simulink model "Vorlage_Gesamtanlage"  (R2022a)
settings: Solver=ode5  StartTime=0.0  StopTime=200  FixedStep=0.01  MaxStep=1  MinStep=0.005  RelTol=1e-3  AbsTol=10  EnableMultiTasking=on
values from neighbouring files (symbols this model uses):
  A = 5    [Parameter.m]
  Flaschengroesse = 10    [Parameter.m]
  I = 0.5    [Parameter.m]
  igetr = 1080    [Parameter.m]
  K = 8    [Parameter.m]
  MaxFlaschen = 25    [Parameter.m]
  MRK = 1    [Parameter.m]
  numA = 0    [Parameter.m]
  PassSilo1 = 1    [Parameter.m]
  PassSilo2 = 1    [Parameter.m]
  PHI = 0.001    [Parameter.m]
  Ra = 40    [Parameter.m]
  SizeSilo1 = 15    [Parameter.m]
  SizeSilo2 = 15    [Parameter.m]
  U = 24    [Parameter.m]
  v_band_abfuhr_set = 2    [Parameter.m]
  v_band_arbeit_set = 30    [Parameter.m]
  v_band_zufuhr_set = 10    [Parameter.m]
  v_umsetzer_greifer_set = 400    [Parameter.m]
  v_umsetzer_set = 80    [Parameter.m]
  v_ve1_set = 400    [Parameter.m]
  v_ve2_set = 400    [Parameter.m]
undefined symbols (not defined in the file or in its folder): Limits
libraries: simulink x94
(part 3 of 3)

== system Vorlage_Gesamtanlage/Abfüllanlage/Flaschen_data/Flaschenstarter/in_Flaschenzähler ==
  Signal : Inport
  Constant : Constant
  Constant1 : Constant  Value=0
  Logical Operator : Logic  AllPortsSameDT=off
  Memory : Memory
  Memory1 : Memory
  Relational Operator : RelationalOperator  Operator===  InputSameDT=off
  Relational Operator1 : RelationalOperator  Operator===  InputSameDT=off
  Sum : Sum  Inputs=|++  OutDataTypeStr=uint16  SaturateOnIntegerOverflow=on
  Rising Edge : Outport
  Count : Outport  Port=2
  wires:
  Signal/1 -> Memory/1, Relational Operator/2
  Constant/1 -> Relational Operator/1
  Relational Operator/1 -> Logical Operator/1
  Constant1/1 -> Relational Operator1/2
  Memory/1 -> Relational Operator1/1
  Relational Operator1/1 -> Logical Operator/2
  Logical Operator/1 -> Sum/1, Rising Edge/1
  Memory1/1 -> Sum/2
  Sum/1 -> Count/1, Memory1/1

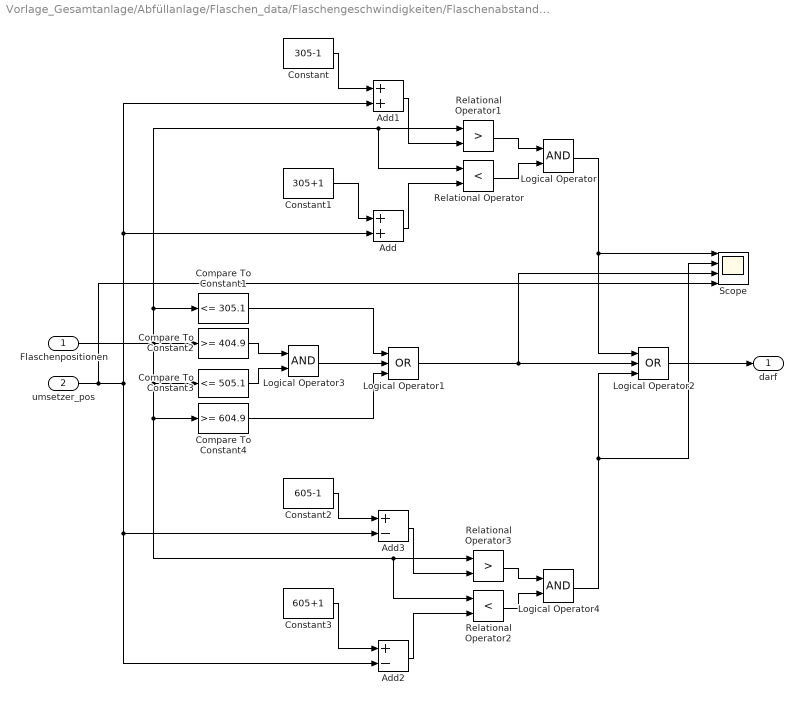
== system Vorlage_Gesamtanlage/Abfüllanlage/Flaschen_data/Flaschengeschwindigkeiten/Flaschenabstandsüberwachung/Umsetzer darf mitnehmen ==
  Flaschenpositionen : Inport
  umsetzer_pos : Inport  Port=2
  Add : Sum
  Add1 : Sum
  Add2 : Sum  Inputs=+-
  Add3 : Sum  Inputs=+-
  Compare To Constant1 : simulink/Logic and Bit Operations/Compare To Constant  relop=<=  const=305.1  OutDataTypeStr=uint8  ZeroCross=off
  Compare To Constant2 : simulink/Logic and Bit Operations/Compare To Constant  relop=>=  const=404.9  OutDataTypeStr=uint8  ZeroCross=off
  Compare To Constant3 : simulink/Logic and Bit Operations/Compare To Constant  relop=<=  const=505.1  OutDataTypeStr=uint8  ZeroCross=off
  Compare To Constant4 : simulink/Logic and Bit Operations/Compare To Constant  relop=>=  const=604.9  OutDataTypeStr=uint8  ZeroCross=off
  Constant : Constant  Value=305-1
  Constant1 : Constant  Value=305+1
  Constant2 : Constant  Value=605-1
  Constant3 : Constant  Value=605+1
  Logical Operator : Logic  AllPortsSameDT=off  OutDataTypeStr=boolean
  Logical Operator1 : Logic  Operator=OR  Inputs=3  AllPortsSameDT=off  OutDataTypeStr=boolean
  Logical Operator2 : Logic  Operator=OR  Inputs=3  AllPortsSameDT=off  OutDataTypeStr=boolean
  Logical Operator3 : Logic  AllPortsSameDT=off  OutDataTypeStr=boolean
  Logical Operator4 : Logic  AllPortsSameDT=off  OutDataTypeStr=boolean
  Relational Operator : RelationalOperator  Operator=<  OutDataTypeStr=boolean  InputSameDT=off
  Relational Operator1 : RelationalOperator  Operator=>  OutDataTypeStr=boolean  InputSameDT=off
  Relational Operator2 : RelationalOperator  Operator=<  OutDataTypeStr=boolean  InputSameDT=off
  Relational Operator3 : RelationalOperator  Operator=>  OutDataTypeStr=boolean  InputSameDT=off
  Scope : Scope  NumInputPorts=4
  darf : Outport
  wires:
  Logical Operator2/1 -> darf/1
  Logical Operator1/1 -> Logical Operator2/2, Scope/3
  Compare To Constant1/1 -> Logical Operator1/1
  Logical Operator/1 -> Logical Operator2/1, Scope/1
  Constant/1 -> Add1/1
  Add1/1 -> Relational Operator1/2
  Relational Operator1/1 -> Logical Operator/1
  Relational Operator/1 -> Logical Operator/2
  Add/1 -> Relational Operator/2
  Constant1/1 -> Add/1
  Compare To Constant2/1 -> Logical Operator3/1
  Compare To Constant3/1 -> Logical Operator3/2
  Logical Operator3/1 -> Logical Operator1/2
  Compare To Constant4/1 -> Logical Operator1/3
  Logical Operator4/1 -> Logical Operator2/3, Scope/2
  Constant2/1 -> Add3/1
  Add3/1 -> Relational Operator3/2
  Relational Operator3/1 -> Logical Operator4/1
  Relational Operator2/1 -> Logical Operator4/2
  Add2/1 -> Relational Operator2/2
  Constant3/1 -> Add2/1
  umsetzer_pos/1 -> Add2/2, Add3/2, Add/2, Add1/2, Scope/4
  Flaschenpositionen/1 -> Compare To Constant2/1, Compare To Constant3/1, Compare To Constant4/1, Relational Operator3/1, Relational Operator2/1, Compare To Constant1/1, Relational Operator1/1, Relational Operator/1

== stateflow chart Vorlage_Gesamtanlage/Abfüllanlage/Drehscheibe/Sensor ==
  state Start
    en: beep = 0;
  state Beep
    en: beep=1;
  (default) -> Start
  Start -> Beep : [ml.mod(winkel, 90) <=2 | ml.mod(winkel, 90) >=88]
  Beep -> Start : [ml.mod(winkel, 90) >2 && ml.mod(winkel, 90) <88]
  data: winkel input double; beep output boolean

== stateflow chart Vorlage_Gesamtanlage/Abfüllanlage/Fehlererkennung/Volle Flasche zum Teller zurück/Chart ==
  state Greife_Flasche_Teller
    entry: error = 0;
  state Oeffne_Greifer_Band
  state Warte_auf_VE2
  state Volle_Flasche_gegriffen
  state Greifer_gestartet
    entry: error = 1;
  state Flasche_weg
  (default) -> Greife_Flasche_Teller
  Flasche_weg -> Greife_Flasche_Teller
  Greife_Flasche_Teller -> Oeffne_Greifer_Band : [I_teller_behaelter_hinten == 1 && i_greifer_zu == 1 && i_umsetz_teller == 1]
  Oeffne_Greifer_Band -> Warte_auf_VE2 : [i_greifer_auf == 1 && i_umsetz_band == 1]
  Volle_Flasche_gegriffen -> Greifer_gestartet [order 1] : [o_umsetz_teller==1]
  Warte_auf_VE2 -> Volle_Flasche_gegriffen [order 2] : [i_greifer_zu == 1]
  Warte_auf_VE2 -> Flasche_weg [order 1] : [i_ve2_herein == 1]
  Volle_Flasche_gegriffen -> Flasche_weg [order 2] : after(5,sec)
  data: I_teller_behaelter_hinten input; i_greifer_zu input; i_umsetz_teller input; i_greifer_auf input; i_umsetz_band input; i_ve2_herein input; error output; o_umsetz_teller input

== stateflow chart Vorlage_Gesamtanlage/Steuerung ==
  state Intelligenz [parallel]
    settings: executionOrder=1
    state Flasche_bewegen [parallel]
      settings: executionOrder=1
      state Initiation
      state Baender_an
        en: send(Arbeitsband_an,Baender);
      state Leere_Flasche_loslassen
        en: send(ums_greifer_auf,Umsetzer)
      state Leere_Flasche_greifen
        en: send(ums_Flasche_greifen,Umsetzer)
      state Umsetzer_zu_Band
        en: send(ums_zu_band,Umsetzer);
      state Leere_Flasche_zu_Teller_umsetzen
        en: send(ums_zu_teller,Umsetzer)
      state Vereineinzeler_1_oeffnen
        en: send(ve1_oeffnen,VE1_2)
        %Dann Leere Flasche durchgehen
      state Leere_Flasche_befuellen
        en: send(silos_oeffnen,Silos)
      state Gefuellte_Flasche_greifen
        en: send(ums_Flasche_greifen,Umsetzer)
      state Gefuellte_Flasche_zu_Band_umsetzen
        en: send(ums_zu_band,Umsetzer)
      state Gefuellte_Flasche_loslassen
        en: send(ums_greifer_auf,Umsetzer)
      state Vereinzeler_2_oeffnen
        en: send(ve2_oeffnen,VE1_2)
        %Dann Gefuellte Flasche weggehne
      state Teller_drehen
        en: send(teller_drehen,Teller)
      state Teller_ausgerichtet
        en: send(teller_ausg,Teller)
        en: send(check,Flasche_voll_check)
      (default) -> Intelligenz.Flasche_bewegen.Initiation
      Intelligenz.Flasche_bewegen.Initiation -> Baender_an
      Baender_an -> Intelligenz.Flasche_bewegen.Umsetzer_zu_Band : [i_umsetzer[3] == 1]
      Intelligenz.Flasche_bewegen.Teller_ausgerichtet -> Intelligenz.Flasche_bewegen.Umsetzer_zu_Band [order 1] : [i_silo[2] == 0 && i_teller[2] == 0]
      Intelligenz.Flasche_bewegen.Leere_Flasche_greifen -> Leere_Flasche_zu_Teller_umsetzen : [i_umsetzer[4] == 1]
      Vereineinzeler_1_oeffnen -> Intelligenz.Flasche_bewegen.Leere_Flasche_greifen : [i_vereinzeler[6] == 1]
      Leere_Flasche_zu_Teller_umsetzen -> Leere_Flasche_loslassen : [i_umsetzer[2] == 1]
      Intelligenz.Flasche_bewegen.Umsetzer_zu_Band -> Vereineinzeler_1_oeffnen : [i_vereinzeler[5] == 1 && i_vereinzeler[6] == 0 && i_teller[2] == 0 && i_umsetzer[1] == 1]
      Vereinzeler_2_oeffnen -> Leere_Flasche_zu_Teller_umsetzen [order 1] : [i_silo[2] == 1 && i_vereinzeler[5] == 0]
      Leere_Flasche_loslassen -> Teller_drehen : [i_umsetzer[3] == 1 && clock - tic > 2 && silo_ventil == 0]
      Vereinzeler_2_oeffnen -> Vereineinzeler_1_oeffnen [order 2] : [i_vereinzeler[4] == 1 && i_vereinzeler[5] == 1]
      Leere_Flasche_befuellen -> Intelligenz.Flasche_bewegen.Umsetzer_zu_Band [order 2] : after(2,sec)[i_teller[2] == 0 ]%Nach Befuellen warten 2s.
      Leere_Flasche_befuellen -> Intelligenz.Flasche_bewegen.Gefuellte_Flasche_greifen [order 1] : after(2,sec)[i_teller[2] == 1]%Nach Befuellen warten 2s.
      Intelligenz.Flasche_bewegen.Teller_ausgerichtet -> Leere_Flasche_befuellen [order 2] : [i_silo[2] == 1 &&( i_silo[3] == 0 && i_silo[4] == 0)]
      Gefuellte_Flasche_loslassen -> Vereinzeler_2_oeffnen : [i_umsetzer[3] == 1 && i_vereinzeler[6] == 1]
      Intelligenz.Flasche_bewegen.Gefuellte_Flasche_greifen -> Gefuellte_Flasche_zu_Band_umsetzen : [i_umsetzer[4] == 1]
      Gefuellte_Flasche_zu_Band_umsetzen -> Gefuellte_Flasche_loslassen : [i_umsetzer[1] == 1]
      Intelligenz.Flasche_bewegen.Teller_ausgerichtet -> Intelligenz.Flasche_bewegen.Gefuellte_Flasche_greifen [order 3] : [i_silo[2] == 0 && i_teller[2] == 1]
      Teller_drehen -> Intelligenz.Flasche_bewegen.Teller_ausgerichtet : after(0.5,sec)[i_teller[1] == 1]
    state Flasche_voll_check [parallel]
      settings: executionOrder=2
      state Initiation
      state check
      state Befuellvorgang_beenden
        en: send(silos_schliessen,Silos)
      (default) -> Intelligenz.Flasche_voll_check.Initiation
      Intelligenz.Flasche_voll_check.Initiation -> check : check
      Befuellvorgang_beenden -> Intelligenz.Flasche_voll_check.Initiation
      check -> Befuellvorgang_beenden : [i_silo[1] == 0]{tic = clock;}
  state Umsetzer [parallel]
    settings: executionOrder=2
    state Leere_Flasche_greifen
      en: o_umsetzer[3] = 0;
      en: o_umsetzer[4] = 1;
    state Greifer_auf_am_Teller
      en: o_umsetzer[4] = 0;
      en: o_umsetzer[3] = 1;
    state Initiation
      en: o_umsetzer[1] = 0;
      en: o_umsetzer[2] = 0;
      en: o_umsetzer[3] = 1;
      en: o_umsetzer[4] = 0;
      %Greifer
    state Leere_Flasche_zu_Teller
      en: o_umsetzer[2] = 1;
      ex: o_umsetzer[2] = 0;
    state Umsetzer_zu_Band
      en: o_umsetzer[1] = 1;
      en: o_umsetzer[3] = 0;
      ex: o_umsetzer[1] = 0;
    note: Da die Anfangsposition des Umsetzers am Teller und Greifer geschlossen ist.
        | Nach der Initiation öffnet er zuerst den Greifer und dann bewegt sich auf das Band zu.
    state Greifer_auf_am_Band
      en: o_umsetzer[4] = 0;
      en: o_umsetzer[3] = 1;
    state Umsetzer_zu_Band_mit_Flasche
      en: o_umsetzer[1] = 1;
      ex: o_umsetzer[1] = 0;
    state Gefuellte_Flasche_greifen
      en: o_umsetzer[4] = 1;
      en: o_umsetzer[3] = 0;
    Greifer_auf_am_Teller -> Umsetzer.Umsetzer_zu_Band [order 2] : ums_zu_band
    (default) -> Umsetzer.Initiation
    Umsetzer.Umsetzer_zu_Band -> Umsetzer.Leere_Flasche_greifen : ums_Flasche_greifen
    Umsetzer.Leere_Flasche_greifen -> Leere_Flasche_zu_Teller : ums_zu_teller
    Umsetzer.Initiation -> Umsetzer.Umsetzer_zu_Band : ums_zu_band
    Leere_Flasche_zu_Teller -> Greifer_auf_am_Teller : ums_greifer_auf
    Greifer_auf_am_Band -> Leere_Flasche_zu_Teller [order 2] : ums_zu_teller
    Greifer_auf_am_Teller -> Umsetzer.Gefuellte_Flasche_greifen [order 1] : ums_Flasche_greifen
    Greifer_auf_am_Band -> Umsetzer.Leere_Flasche_greifen [order 1] : ums_Flasche_greifen
    Umsetzer_zu_Band_mit_Flasche -> Greifer_auf_am_Band : ums_greifer_auf
    Umsetzer.Gefuellte_Flasche_greifen -> Umsetzer_zu_Band_mit_Flasche : ums_zu_band
  state Baender [parallel]
    settings: executionOrder=3
    state Initiation
      en:o_band[1] = 1;
      %Zufuhrband an
      en:o_band[2] = 0;
      %Arbeitsband aus
    state Arbeitsband_an
      en:o_band[2]=1;
    (default) -> Baender.Initiation
    Baender.Initiation -> Arbeitsband_an : Arbeitsband_an [i_band==1]
  state Silos [parallel]
    settings: executionOrder=4
    state Initiation
      en: o_silo[1] = 0;
      en: o_silo[2] = 0;
      en: silo_ventil = 0;
      %Silo geschlossen
    state Silos_oeffnen
      en: o_silo[1] = 1;
      en: o_silo[2] = 1;
      en: silo_ventil = 1;
    (default) -> Silos.Initiation
    Silos.Initiation -> Silos_oeffnen : silos_oeffnen
    Silos_oeffnen -> Silos.Initiation : silos_schliessen
  state VE1_2 [parallel]
    settings: executionOrder=5
    state init
      en: o_vereinzeler[1] = 0;
      en: o_vereinzeler[2] = 0;
    state ve1_oeffnen
      en: o_vereinzeler[1]  = 1;
    state ve1_schliessen
      en: o_vereinzeler[1] = 0;
    state ve2_schliessen
      en: o_vereinzeler[2] = 0;
    state ve2_oeffnen
      en: o_vereinzeler[2] = 1;
    (default) -> init
    init -> ve1_oeffnen : ve1_oeffnen
    ve1_schliessen -> ve1_oeffnen [order 1] : ve1_oeffnen
    ve1_oeffnen -> ve1_schliessen : after(1,sec)
    ve1_schliessen -> ve2_oeffnen [order 2] : ve2_oeffnen
    ve2_schliessen -> ve1_oeffnen [order 1] : ve1_oeffnen
    ve2_oeffnen -> ve2_schliessen : after(1,sec)
    ve2_schliessen -> ve2_oeffnen [order 2] : ve2_oeffnen
  state Teller [parallel]
    settings: executionOrder=6
    state Teller_Drehen
      en: o_teller = 1;
    state Initiation
      en: o_teller = 1;
    state Teller_ausgerichtet
      en: o_teller = 0;
    (default) -> Teller.Initiation
    Teller.Teller_ausgerichtet -> Teller_Drehen : teller_drehen
    Teller.Initiation -> Teller.Teller_ausgerichtet : [i_teller[1] == 1]
    Teller_Drehen -> Teller.Teller_ausgerichtet : teller_ausg
  data: i_band input boolean; o_band output double size=2; o_vereinzeler output double size=2; o_silo output double size=2; o_umsetzer output double size=4; o_teller output double; i_vereinzeler input boolean size=6; i_silo input boolean size=4; i_umsetzer input boolean size=4; i_teller input boolean size=2; clock input double; tic local double; silo_ventil local double
  events: ums_zu_band local FUNCTION_CALL_EVENT; ve1_oeffnen local FUNCTION_CALL_EVENT; ums_Flasche_greifen local FUNCTION_CALL_EVENT; ums_zu_teller local FUNCTION_CALL_EVENT; ums_greifer_auf local FUNCTION_CALL_EVENT; teller_drehen local FUNCTION_CALL_EVENT; silos_oeffnen local FUNCTION_CALL_EVENT; silos_schliessen local FUNCTION_CALL_EVENT; ve2_oeffnen local FUNCTION_CALL_EVENT; Arbeitsband_an local FUNCTION_CALL_EVENT; check local FUNCTION_CALL_EVENT; teller_ausg local FUNCTION_CALL_EVENT
